simulink subsystem "rss_FaltLevlCmpt"  (R2023a)
settings: Solver=VariableStepAuto  StartTime=0.0  StopTime=10.0  RelTol=1e-3
undefined symbols (not defined in the file): Cdbl_numFaltDiaNum
settings Model: Creator=xiaoqiang.yuan  LastModifiedBy=xiaoqiang.yuan

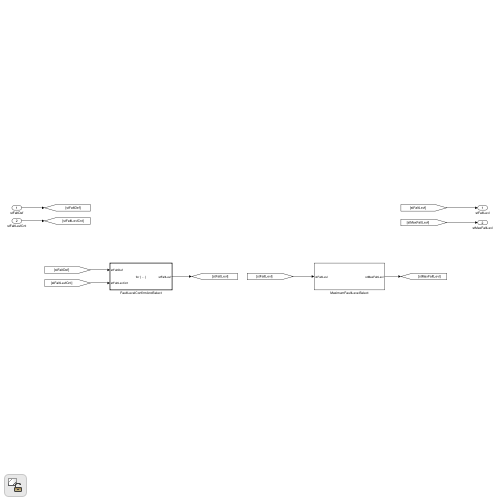
[thumbnail: Simulink's stored preview of the top-level diagram]
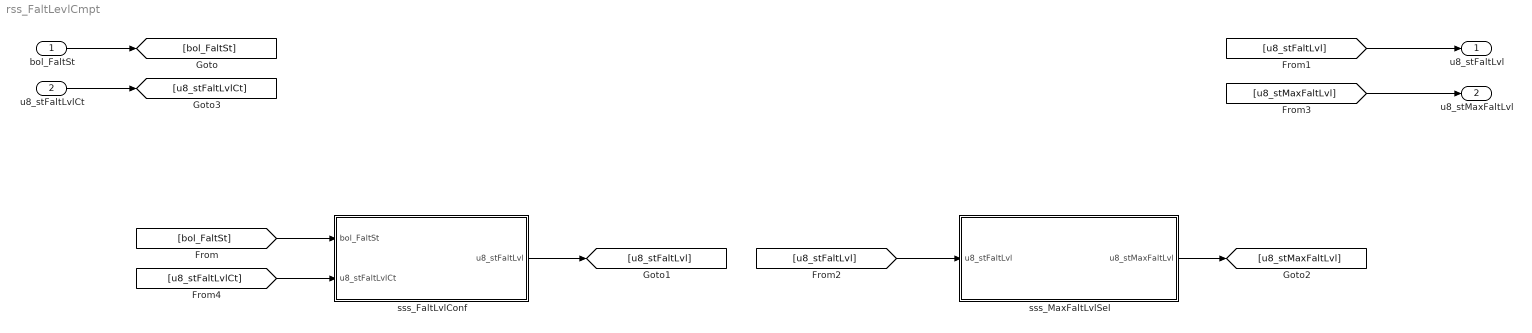
== system rss_FaltLevlCmpt ==
  bol_FaltSt : Inport  OutDataTypeStr=boolean
  u8_stFaltLvlCt : Inport  Port=2  OutDataTypeStr=uint8
  sss_FaltLvlConf : Subsystem  TreatAsAtomicUnit=on
      settings: RTWSystemCode=Nonreusable function
  sss_MaxFaltLvlSel : Subsystem
      settings: RTWSystemCode=Nonreusable function
  u8_stFaltLvl : Outport  OutDataTypeStr=uint8
  u8_stMaxFaltLvl : Outport  Port=2  OutDataTypeStr=uint8
  wires:
  sss_FaltLvlConf/1(u8_stFaltLvl) -> [u8_stFaltLvl]
  [bol_FaltSt] -> sss_FaltLvlConf/1(bol_FaltSt)
  bol_FaltSt/1 -> [bol_FaltSt]
  [u8_stFaltLvl] -> u8_stFaltLvl/1
  [u8_stFaltLvl] -> sss_MaxFaltLvlSel/1(u8_stFaltLvl)
  [u8_stMaxFaltLvl] -> u8_stMaxFaltLvl/1
  sss_MaxFaltLvlSel/1(u8_stMaxFaltLvl) -> [u8_stMaxFaltLvl]
  u8_stFaltLvlCt/1 -> [u8_stFaltLvlCt]
  [u8_stFaltLvlCt] -> sss_FaltLvlConf/2(u8_stFaltLvlCt)

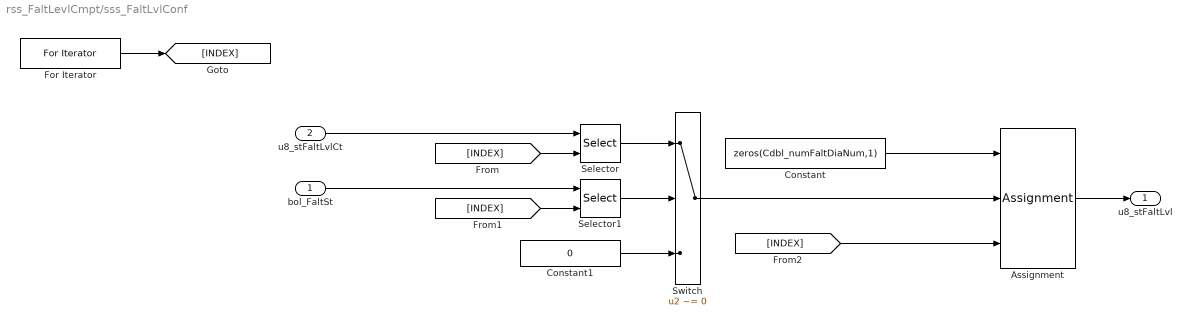
== system rss_FaltLevlCmpt/sss_FaltLvlConf ==
  bol_FaltSt : Inport
  u8_stFaltLvlCt : Inport  Port=2
  Assignment : Assignment  DiagnosticForDimensions=Warning  IndexOptions=Index vector (port)  Indices=1  OutputSizes=1
  Constant : Constant  Value=zeros(Cdbl_numFaltDiaNum,1)  OutDataTypeStr=uint8
  Constant1 : Constant  Value=0  OutDataTypeStr=uint8
  For Iterator : ForIterator  IterationLimit=Cdbl_numFaltDiaNum  IterationVariableDataType=uint8
  Selector : Selector  InputPortWidth=Cdbl_numFaltDiaNum  IndexOptions=Index vector (port)  Indices=[1 3]  OutputSizes=1
  Selector1 : Selector  InputPortWidth=Cdbl_numFaltDiaNum  IndexOptions=Index vector (port)  Indices=[1 3]  OutputSizes=1
  Switch : Switch  Criteria=u2 ~= 0  SaturateOnIntegerOverflow=off  InputSameDT=off
  u8_stFaltLvl : Outport
  wires:
  Assignment/1 -> u8_stFaltLvl/1
  Constant/1 -> Assignment/1
  Selector/1 -> Switch/1
  Constant1/1 -> Switch/3
  u8_stFaltLvlCt/1 -> Selector/1
  bol_FaltSt/1 -> Selector1/1
  For Iterator/1 -> [INDEX]
  [INDEX] -> Selector/2
  [INDEX] -> Selector1/2
  Selector1/1 -> Switch/2
  Switch/1 -> Assignment/2
  [INDEX] -> Assignment/3

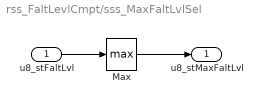
== system rss_FaltLevlCmpt/sss_MaxFaltLvlSel ==
  u8_stFaltLvl : Inport
  Max : MinMax  Function=max
  u8_stMaxFaltLvl : Outport
  wires:
  Max/1 -> u8_stMaxFaltLvl/1
  u8_stFaltLvl/1 -> Max/1
